simulink model "motor1"  (R2022b)
settings: Solver=FixedStepDiscrete  StartTime=0.0  StopTime=6  FixedStep=sys.Ts  MaxStep=0.0001  RelTol=1e-3
undefined symbols (not defined in the file or in its folder): awu, dac, degs2rpm, dend, DiscIntNeverNeededParam, National_Instruments, numd, PCIe, pid, rpm2rads, sens, step, sys
libraries: sldrtlib x3
settings Model: SimulationMode=external  ExtModeTrigDuration=10000  Creator=loren  LastModifiedBy=francesch2
settings DataIOCC: ReturnWorkspaceOutputs=off
settings HardwareCC: ProdBitPerLong=64  ProdHWDeviceType=Intel->x86-64 (Linux 64)
settings ModelReferenceCC: EnableRefExpFcnMdlSchedulingChecks=on
settings RTWCC: Description=Simulink Desktop Real-Time  SystemTargetFile=sldrt.tlc  TemplateMakefile=sldrt.tmf  RTWCompilerOptimization=on
settings CodeAppCC: MaxIdLength=95
settings SimulinkDesktopRealTimeCC: TargetLibSuffix=_sldrt.a  TargetPreCompLibLocation=C:\Program Files\MATLAB\R2022b\toolbox\sldrt\lib\win64

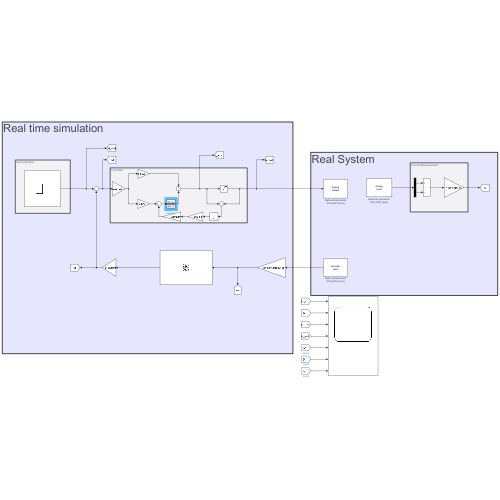
[thumbnail: Simulink's stored preview of the top-level diagram]
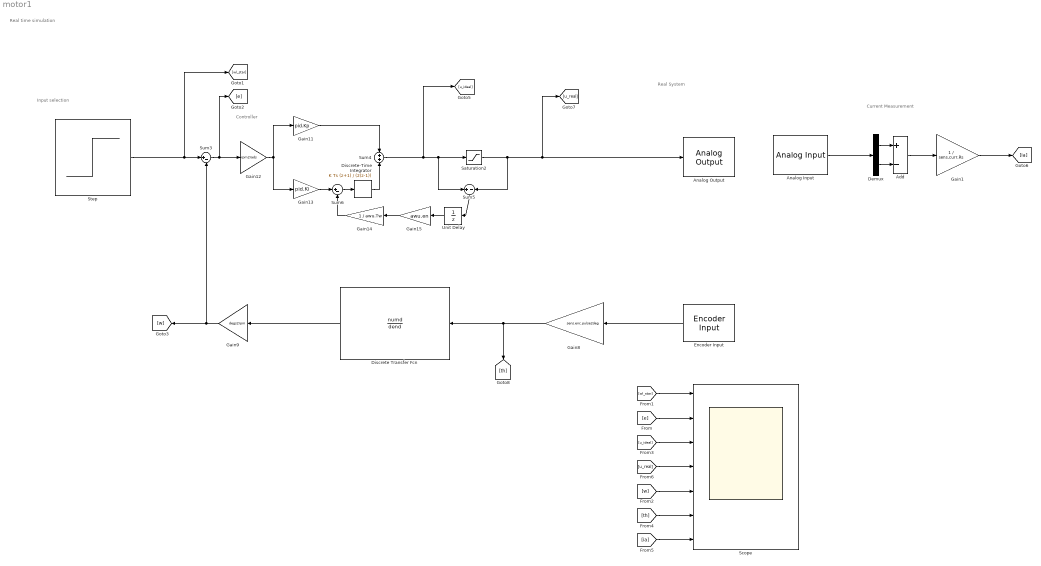
== system motor1 ==
  note: Real time simulation
  note: Input selection
  note: Controller
  note: Real System
  note: Current Measurement
  Add : Sum  Inputs=+-
  Analog Input : sldrtlib/Analog Input  SampleTime=-1  MaxMissedTicks=10  ShowMissedTicks=off  YieldWhenWaiting=off  DrvName=National_Instruments/PCIe-6321  DrvAddress=4294967295  DrvOptions=[0 0 0 2 0 0 0]  Channels=[1 2]  RangeMode=1  VoltRange=1  DataType=1
      settings: AttributesFormatString=National Instruments\nPCIe-6321 [auto]
  Analog Output : sldrtlib/Analog Output  SampleTime=-1  MaxMissedTicks=10  ShowMissedTicks=off  YieldWhenWaiting=off  DrvName=National_Instruments/PCIe-6321  DrvAddress=4294967295  DrvOptions=[0 0 0 2 0 0 0]  Channels=1  RangeMode=1  VoltRange=1  InitialValue=0  FinalValue=0
      settings: AttributesFormatString=National Instruments\nPCIe-6321 [auto]
  Demux : Demux  Outputs=2
  Discrete Transfer Fcn : DiscreteTransferFcn  Numerator=numd  Denominator=dend  SampleTime=sys.Ts
  Discrete-Time Integrator : DiscreteIntegrator  IntegratorMethod=Integration: Trapezoidal  SampleTime=sys.Ts  ICPrevOutput=DiscIntNeverNeededParam  ICPrevScaledInput=DiscIntNeverNeededParam
  Encoder Input : sldrtlib/Encoder Input  SampleTime=-1  MaxMissedTicks=10  ShowMissedTicks=off  YieldWhenWaiting=off  DrvName=National_Instruments/PCIe-6321  DrvAddress=4294967295  DrvOptions=[0 0 0 2 0 0 0]  Channels=1  QuadMode=3  IndexPulse=1  InputFilter=Inf  DataType=1
      settings: AttributesFormatString=National Instruments\nPCIe-6321 [auto]
  Gain1 : Gain  Gain=1 / sens.curr.Rs
  Gain11 : Gain  Gain=pid.Kp
  Gain12 : Gain  Gain=rpm2rads
  Gain13 : Gain  Gain=pid.Ki
  Gain14 : Gain  Gain=1 / awu.Tw
  Gain15 : Gain  Gain=awu.en
  Gain8 : Gain  Gain=sens.enc.pulse2deg
  Gain9 : Gain  Gain=degs2rpm
  Saturation2 : Saturate  UpperLimit=dac.V  LowerLimit=-dac.V
  Scope : Scope  NumInputPorts=7
  Step : Step  Time=step.t  After=step.A  SampleTime=0
  Sum3 : Sum  Inputs=|+-
  Sum4 : Sum  Inputs=+|+
  Sum5 : Sum  Inputs=+|-
  Sum6 : Sum  Inputs=|+-
  Unit Delay : UnitDelay  SampleTime=-1  HasFrameUpgradeWarning=on
  wires:
  Gain9/1 -> [w], Sum3/2
  Sum3/1 -> [e], Gain12/1
  Gain12/1 -> Gain13/1, Gain11/1
  Sum4/1 -> [u_ideal], Saturation2/1, Sum5/1
  Gain11/1 -> Sum4/1
  Discrete-Time Integrator/1 -> Sum4/2
  Step/1 -> [wl_star], Sum3/1
  Gain13/1 -> Sum6/1
  Sum6/1 -> Discrete-Time Integrator/1
  Saturation2/1 -> Sum5/2, [u_real], Analog Output/1
  Sum5/1 -> Unit Delay/1
  Gain14/1 -> Sum6/2
  Gain15/1 -> Gain14/1
  Discrete Transfer Fcn/1 -> Gain9/1
  Gain8/1 -> Discrete Transfer Fcn/1, [th]
  Unit Delay/1 -> Gain15/1
  Analog Input/1 -> Demux/1
  Gain1/1 -> [ia]
  Demux/1 -> Add/1
  Add/1 -> Gain1/1
  Demux/2 -> Add/2
  Encoder Input/1 -> Gain8/1
  [u_ideal] -> Scope/3
  [e] -> Scope/2
  [w] -> Scope/5
  [wl_star] -> Scope/1
  [th] -> Scope/6
  [u_real] -> Scope/4
  [ia] -> Scope/7
